simulink model "PV_MODULE_CHARACTERISTICS_MODEL"  (R2016b)
settings: Solver=VariableStepAuto  StartTime=0.0  StopTime=0.1  RelTol=1e-3
values from neighbouring files (symbols this model uses):
  A = 1.3    [PV_module_Code.m]
  Isc = 8.61    [PV_module_Code.m]
  Ki = 0.002    [PV_module_Code.m]
  Kv = -0.32    [PV_module_Code.m]
  Ns = 60    [PV_module_Code.m]
  Rp = 415    [PV_module_Code.m]
  Rs = 0.22    [PV_module_Code.m]
  Voc = 37.41    [PV_module_Code.m]
libraries: powerlib x5
settings Model: Creator=adria  LastModifiedBy=adria
settings DebuggingCC: UnconnectedInputMsg=none  UnconnectedOutputMsg=none  UnconnectedLineMsg=none

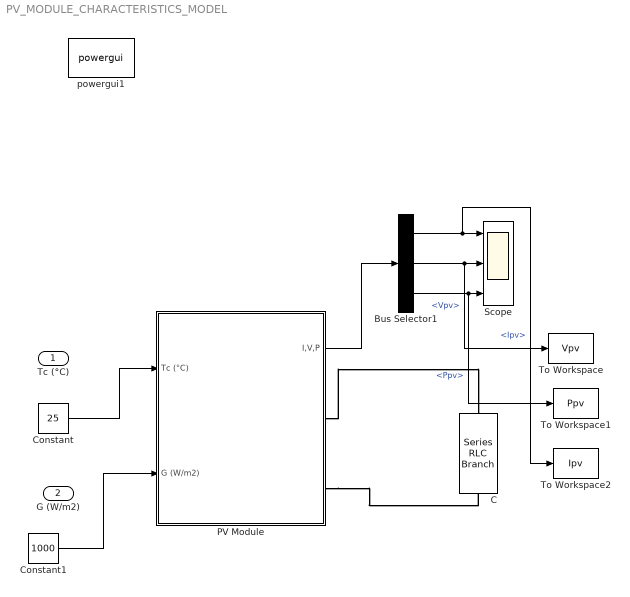
== system PV_MODULE_CHARACTERISTICS_MODEL ==
  Tc (°C) : Inport
  G (W/m2) : Inport  Port=2
  Bus Selector1 : BusSelector  OutputSignals=Ipv,Vpv,Ppv
  C : powerlib/Elements/Series RLC Branch  LConnTagsString=__new0  RConnTagsString=__new0  BranchType=R  Resistance=100  Inductance=1e-3  SetiL0=off  InitialCurrent=0  Capacitance=19e-4  Setx0=off  InitialVoltage=0  Measurements=Branch voltage
  Constant : Constant  Value=25
  Constant1 : Constant  Value=1000
  PV Module : Subsystem
  Scope : Scope  NumInputPorts=3
  To Workspace : ToWorkspace  VariableName=Vpv  SampleTime=-1
  To Workspace1 : ToWorkspace  VariableName=Ppv  SampleTime=-1
  To Workspace2 : ToWorkspace  VariableName=Ipv  SampleTime=-1
  powergui1 : powerlib/powergui  Priority=1  SimulationMode=Discrete  SolverType=Tustin/Backward Euler (TBE)  SampleTime=1e-5  frequency=60  SPID=off  DisableSnubberDevices=off  DisableRonSwitches=off  DisableVfSwitches=off  SwTol=0  DisplayEquations=off  Interpol=off  ExternalGateDelay=off  methode=off  Ts=10  FunctionMessages=off  echomessages=off  HookPort=off  EnableUseOfTLC=off  x0status=blocks  frequencyindice=0  Pbase=100e6  ErrMax=1e-4  Iterations=50  UnitsV=kV  UnitsW=MW  buscounter=0  RestoreLinks=warning  ResistiveCurrentMeasurement=off  Frange=[0:2:500]  Ylog=off  Xlog=on  ShowGrid=off  save=off  variable=ZData  structure=0  ZoomFFT=off  StartTime=0.0  cycles=1  DisplayStyle=1  fundamental=60  FreqAxis=off  MaxFrequency=1000  frequencyindicesteady=1  RmsSteady=1  display=off
  wires:
  PV Module/1(I,V,P) -> Bus Selector1/1
  Constant/1 -> PV Module/1(Tc (°C))
  Constant1/1 -> PV Module/2(G (W/m2))
  Bus Selector1/2 -> To Workspace/1, Scope/2  "<Vpv>"
  Bus Selector1/3 -> To Workspace1/1, Scope/3  "<Ppv>"
  Bus Selector1/1 -> To Workspace2/1, Scope/1  "<Ipv>"
  connections:
  PV Module/RConn1 -- C/LConn1
  PV Module/RConn2 -- C/RConn1

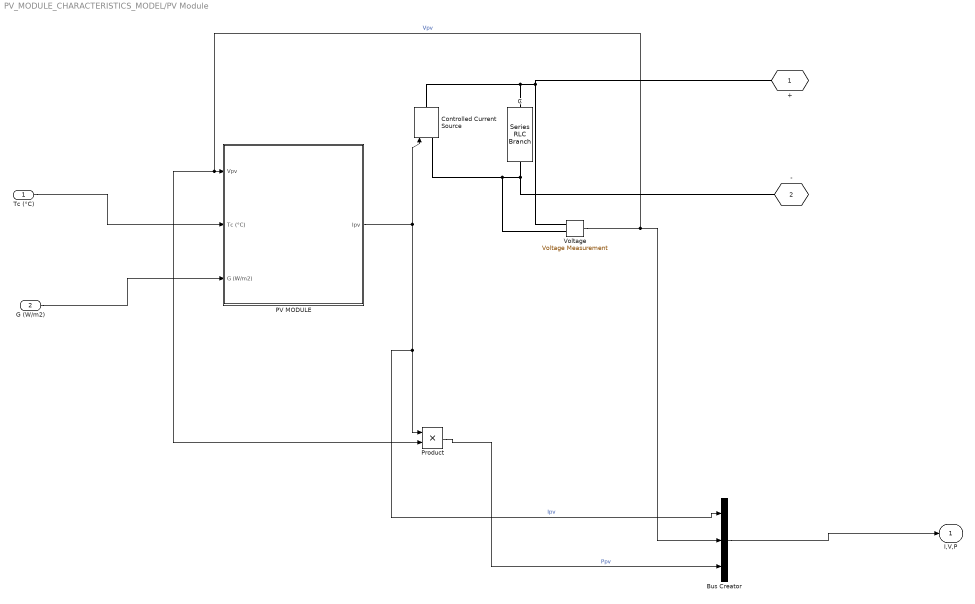
== system PV_MODULE_CHARACTERISTICS_MODEL/PV Module ==
  Tc (°C) : Inport
  G (W/m2) : Inport  Port=2
  Bus Creator : BusCreator  Inputs='Ipv','Vpv','Ppv'
  C : powerlib/Elements/Series RLC Branch  LConnTagsString=__new0  RConnTagsString=__new0  BranchType=C  Resistance=10  Inductance=1e-3  SetiL0=off  InitialCurrent=0  Capacitance=19e-4  Setx0=off  InitialVoltage=0  Measurements=Branch voltage
  Controlled Current Source : powerlib/Electrical Sources/Controlled Current Source  Initialize=on  Source_Type=AC  Amplitude=0  Phase=0  Frequency=0  Measurements=None
  PV MODULE : Subsystem
  Product : Product
  "Voltage " : powerlib/Measurements/Voltage Measurement  PhasorSimulation=off  OutputType=Complex  PSBequivalent=0
  + : PMIOPort  Port=1  Side=Right
  - : PMIOPort  Port=2  Side=Right
  I,V,P : Outport
  wires:
  Product/1 -> Bus Creator/3  "Ppv"
  Tc (°C)/1 -> PV MODULE/2("Tc (°C) ")
  G (W/m2)/1 -> PV MODULE/3(G (W/m2))
  "Voltage "/1 -> Product/2, PV MODULE/1(Vpv), Bus Creator/2  "Vpv"
  PV MODULE/1(Ipv) -> Controlled Current Source/1, Bus Creator/1, Product/1  "Ipv"
  Bus Creator/1 -> I,V,P/1
  connections:
  Controlled Current Source/LConn1 -- -/RConn1 -- C/RConn1 -- "Voltage "/LConn2
  Controlled Current Source/RConn1 -- C/LConn1 -- +/RConn1 -- "Voltage "/LConn1

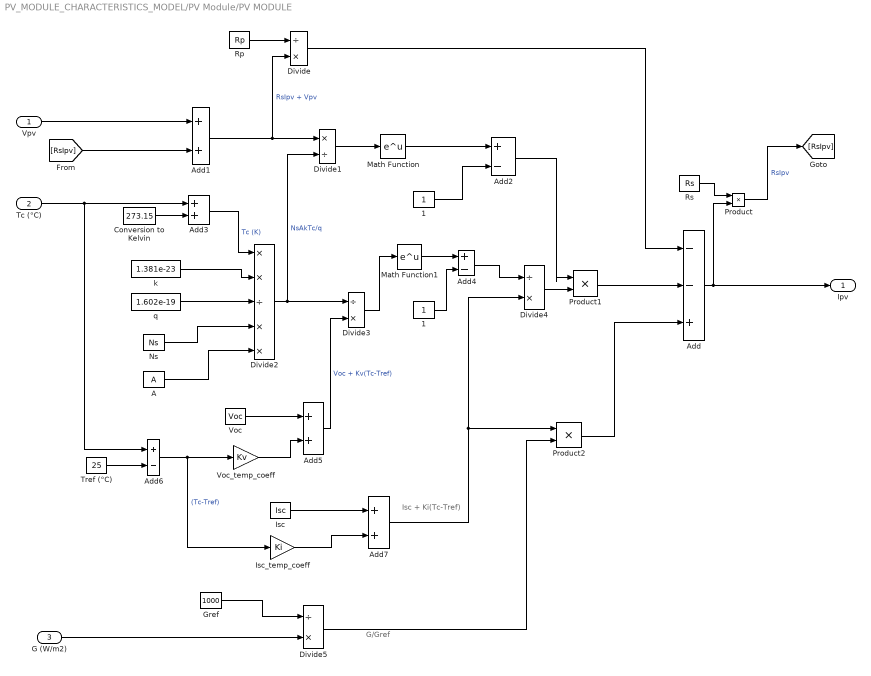
== system PV_MODULE_CHARACTERISTICS_MODEL/PV Module/PV MODULE ==
  note: G/Gref
  note: Isc + Ki(Tc-Tref)
  Vpv : Inport
  "Tc (°C) " : Inport  Port=2
  G (W/m2) : Inport  Port=3
  " 1" : Constant
  " Gref " : Constant  Value=1000
  " Tref (°C)" : Constant  Value=25
  " Voc" : Constant  Value=Voc
  1 : Constant
  A : Constant  Value=A
  Add : Sum  Inputs=--+
  Add{1,3,5,7} (4 alike) : Sum
  Add2 : Sum  Inputs=+-
  Add4 : Sum  Inputs=+-
  Add6 : Sum  Inputs=+-
  Conversion to Kelvin : Constant  Value=273.15
  Divide{,3..5} (4 alike) : Product  Inputs=/*
  Divide1 : Product  Inputs=*/
  Divide2 : Product  Inputs=**/**
  Isc : Constant  Value=Isc
  "Isc_temp_coeff " : Gain  Gain=Ki
  Math Function : Math  SaturateOnIntegerOverflow=on
  Math Function1 : Math  SaturateOnIntegerOverflow=on
  Ns : Constant  Value=Ns
  Product : Product
  Product1 : Product
  Product2 : Product
  Rp : Constant  Value=Rp
  Rs : Constant  Value=Rs
  Voc_temp_coeff : Gain  Gain=Kv
  k : Constant  Value=1.381e-23
  "q " : Constant  Value=1.602e-19
  Ipv : Outport
  wires:
  A/1 -> Divide2/5
  Vpv/1 -> Add1/1
  Rp/1 -> Divide/1
  Add/1 -> Ipv/1, Product/2
  Product/1 -> [RsIpv]  "RsIpv"
  Divide/1 -> Add/1
  Add1/1 -> Divide1/1, Divide/2  "RsIpv + Vpv"
  Rs/1 -> Product/1
  Product2/1 -> Add/3
  Divide2/1 -> Divide3/1, Divide1/2  "NsAkTc/q"
  k/1 -> Divide2/2
  Math Function1/1 -> Add4/1
  " Voc"/1 -> Add5/1
  Divide4/1 -> Product1/2
  Add2/1 -> Product1/1
  Math Function/1 -> Add2/1
  Divide3/1 -> Math Function1/1
  "q "/1 -> Divide2/3
  Add6/1 -> "Isc_temp_coeff "/1, Voc_temp_coeff/1  "(Tc-Tref)"
  " 1"/1 -> Add4/2
  Isc/1 -> Add7/1
  Add7/1 -> Product2/1, Divide4/2
  "Tc (°C) "/1 -> Add6/1, Add3/1
  Add4/1 -> Divide4/1
  Product1/1 -> Add/2
  Divide5/1 -> Product2/2
  Conversion to Kelvin/1 -> Add3/2
  Add5/1 -> Divide3/2  "Voc + Kv(Tc-Tref)"
  "Isc_temp_coeff "/1 -> Add7/2
  Divide1/1 -> Math Function/1
  " Gref "/1 -> Divide5/1
  " Tref (°C)"/1 -> Add6/2
  G (W/m2)/1 -> Divide5/2
  Voc_temp_coeff/1 -> Add5/2
  Add3/1 -> Divide2/1  "Tc (K)"
  Ns/1 -> Divide2/4
  1/1 -> Add2/2
  [RsIpv] -> Add1/2
